simulink model "TST_CrCtl_Governor"  (R2016b)
settings: Solver=FixedStepDiscrete  StartTime=0.0  StopTime=simTime  FixedStep=sampleTime  RelTol=1e-3
values from neighbouring files (symbols this model uses):
  testCase = 1    [initTST_CrCtl_Governor_001.m]    (also in initTST_CrCtl_Governor_002.m = 2; initTST_CrCtl_Governor_003.m = 3; initTST_CrCtl_Governor_004.m = 4; initTST_CrCtl_Governor_005.m = 5)
libraries: simulink x144, UnitTest_Lib x110
(part 1 of 7)
settings Model: Creator=guanxiaoxing  LastModifiedBy=guanxiaoxing
settings DebuggingCC: SignalRangeChecking=error

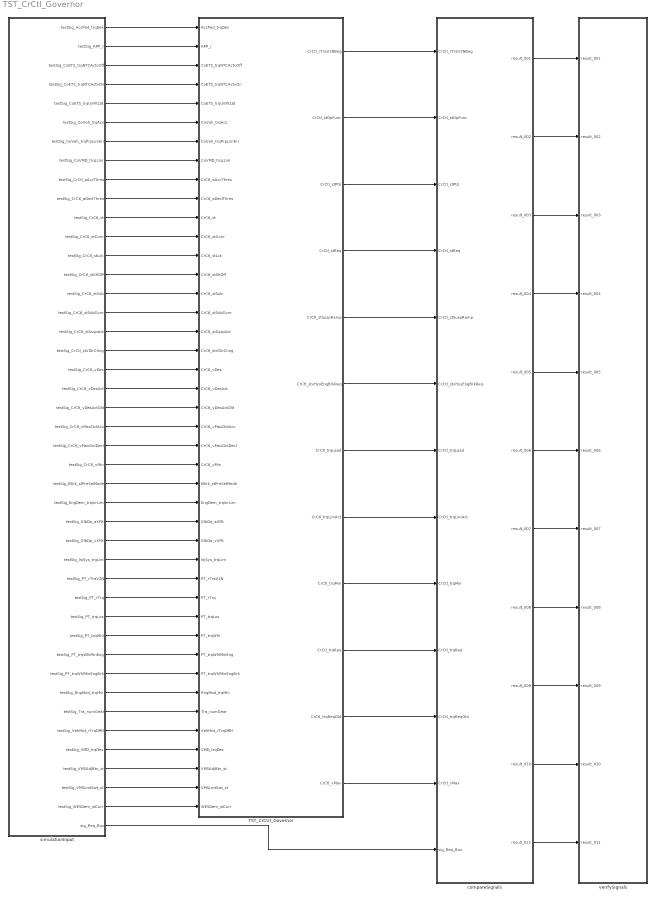
== system TST_CrCtl_Governor ==
  TST_CrCUI_Governor : Subsystem
  compareSignals : Subsystem
  simulationInput : Subsystem
  verifySignals : Subsystem
  wires:
  simulationInput/1(testSig_AccPed_trqDes) -> TST_CrCUI_Governor/1(AccPed_trqDes)
  simulationInput/2(testSig_APP_r) -> TST_CrCUI_Governor/2(APP_r)
  simulationInput/3(testSig_CoETS_trqNTCActvOff) -> TST_CrCUI_Governor/3(CoETS_trqNTCActvOff)
  simulationInput/4(testSig_CoETS_trqNTCActvOn) -> TST_CrCUI_Governor/4(CoETS_trqNTCActvOn)
  simulationInput/5(testSig_CoETS_trqUnFltLtd) -> TST_CrCUI_Governor/5(CoETS_trqUnFltLtd)
  simulationInput/6(testSig_CoVeh_trqAcs) -> TST_CrCUI_Governor/6(CoVeh_trqAcs)
  simulationInput/7(testSig_CoVeh_trqPrpLimErr) -> TST_CrCUI_Governor/7(CoVeh_trqPrpLimErr)
  simulationInput/8(testSig_CoVMD_trqLLim) -> TST_CrCUI_Governor/8(CoVMD_trqLLim)
  simulationInput/9(testSig_CrCtl_aAccThres) -> TST_CrCUI_Governor/9(CrCtl_aAccThres)
  simulationInput/10(testSig_CrCtl_aDeclThres) -> TST_CrCUI_Governor/10(CrCtl_aDeclThres)
  simulationInput/11(testSig_CrCtl_st) -> TST_CrCUI_Governor/11(CrCtl_st)
  simulationInput/12(testSig_CrCtl_stGvnr) -> TST_CrCUI_Governor/12(CrCtl_stGvnr)
  simulationInput/13(testSig_CrCtl_stLck) -> TST_CrCUI_Governor/13(CrCtl_stLck)
  simulationInput/14(testSig_CrCtl_stShOff) -> TST_CrCUI_Governor/14(CrCtl_stShOff)
  simulationInput/15(testSig_CrCtl_stSub) -> TST_CrCUI_Governor/15(CrCtl_stSub)
  simulationInput/16(testSig_CrCtl_stSubGvnr) -> TST_CrCUI_Governor/16(CrCtl_stSubGvnr)
  simulationInput/17(testSig_CrCtl_stSuspAct) -> TST_CrCUI_Governor/17(CrCtl_stSuspAct)
  simulationInput/18(testSig_CrCtl_stVDirChng) -> TST_CrCUI_Governor/18(CrCtl_stVDirChng)
  simulationInput/19(testSig_CrCtl_vDes) -> TST_CrCUI_Governor/19(CrCtl_vDes)
  simulationInput/20(testSig_CrCtl_vDesAct) -> TST_CrCUI_Governor/20(CrCtl_vDesAct)
  simulationInput/21(testSig_CrCtl_vDesActOld) -> TST_CrCUI_Governor/21(CrCtl_vDesActOld)
  simulationInput/22(testSig_CrCtl_vMaxDvtAcc) -> TST_CrCUI_Governor/22(CrCtl_vMaxDvtAcc)
  simulationInput/23(testSig_CrCtl_vMaxDvtDecl) -> TST_CrCUI_Governor/23(CrCtl_vMaxDvtDecl)
  simulationInput/24(testSig_CrCtl_vMin) -> TST_CrCUI_Governor/24(CrCtl_vMin)
  simulationInput/25(testSig_EBrk_stPreSelMode) -> TST_CrCUI_Governor/25(EBrk_stPreSelMode)
  simulationInput/26(testSig_EngDem_trqInrLim) -> TST_CrCUI_Governor/26(EngDem_trqInrLim)
  simulationInput/27(testSig_GlbDa_aXFlt) -> TST_CrCUI_Governor/27(GlbDa_aXFlt)
  simulationInput/28(testSig_GlbDa_vXFlt) -> TST_CrCUI_Governor/28(GlbDa_vXFlt)
  simulationInput/29(testSig_InjSys_trqLim) -> TST_CrCUI_Governor/29(InjSys_trqLim)
  simulationInput/30(testSig_PT_rTraV2N) -> TST_CrCUI_Governor/30(PT_rTraV2N)
  simulationInput/31(testSig_PT_rTrq) -> TST_CrCUI_Governor/31(PT_rTrq)
  simulationInput/32(testSig_PT_trqLos) -> TST_CrCUI_Governor/32(PT_trqLos)
  simulationInput/33(testSig_PT_trqWhl) -> TST_CrCUI_Governor/33(PT_trqWhl)
  simulationInput/34(testSig_PT_trqWhlMinEng) -> TST_CrCUI_Governor/34(PT_trqWhlMinEng)
  simulationInput/35(testSig_PT_trqWhlMinEngBrk) -> TST_CrCUI_Governor/35(PT_trqWhlMinEngBrk)
  simulationInput/36(testSig_RngMod_trqMin) -> TST_CrCUI_Governor/36(RngMod_trqMin)
  simulationInput/37(testSig_Tra_numGear) -> TST_CrCUI_Governor/37(Tra_numGear)
  simulationInput/38(testSig_VehMot_rTrqDfftl) -> TST_CrCUI_Governor/38(VehMot_rTrqDfftl)
  simulationInput/39(testSig_VMD_trqDes) -> TST_CrCUI_Governor/39(VMD_trqDes)
  simulationInput/40(testSig_VMSAdjBtn_st) -> TST_CrCUI_Governor/40(VMSAdjBtn_st)
  simulationInput/41(testSig_VMSLmtSwt_st) -> TST_CrCUI_Governor/41(VMSLmtSwt_st)
  simulationInput/42(testSig_WESDem_stCurr) -> TST_CrCUI_Governor/42(WESDem_stCurr)
  TST_CrCUI_Governor/1(CrCtl_rTraV2NBeg) -> compareSignals/1(CrCtl_rTraV2NBeg)
  TST_CrCUI_Governor/2(CrCtl_stOpFunc) -> compareSignals/2(CrCtl_stOpFunc)
  TST_CrCUI_Governor/3(CrCtl_stPtd) -> compareSignals/3(CrCtl_stPtd)
  TST_CrCUI_Governor/4(CrCtl_stReq) -> compareSignals/4(CrCtl_stReq)
  TST_CrCUI_Governor/5(CrCtl_stSuspRamp) -> compareSignals/5(CrCtl_stSuspRamp)
  TST_CrCUI_Governor/6(CrCtl_stvHysEngBrkReq) -> compareSignals/6(CrCtl_stvHysEngBrkReq)
  TST_CrCUI_Governor/7(CrCtl_trqLead) -> compareSignals/7(CrCtl_trqLead)
  TST_CrCUI_Governor/8(CrCtl_trqLimAct) -> compareSignals/8(CrCtl_trqLimAct)
  TST_CrCUI_Governor/9(CrCtl_trqMin) -> compareSignals/9(CrCtl_trqMin)
  TST_CrCUI_Governor/10(CrCtl_trqReq) -> compareSignals/10(CrCtl_trqReq)
  TST_CrCUI_Governor/11(CrCtl_trqReqOld) -> compareSignals/11(CrCtl_trqReqOld)
  TST_CrCUI_Governor/12(CrCtl_vMax) -> compareSignals/12(CrCtl_vMax)
  simulationInput/43(sig_Req_Bus) -> compareSignals/13(sig_Req_Bus)
  compareSignals/1(result_001) -> verifySignals/1(result_001)
  compareSignals/2(result_002) -> verifySignals/2(result_002)
  compareSignals/3(result_003) -> verifySignals/3(result_003)
  compareSignals/4(result_004) -> verifySignals/4(result_004)
  compareSignals/5(result_005) -> verifySignals/5(result_005)
  compareSignals/6(result_006) -> verifySignals/6(result_006)
  compareSignals/7(result_007) -> verifySignals/7(result_007)
  compareSignals/8(result_008) -> verifySignals/8(result_008)
  compareSignals/9(result_009) -> verifySignals/9(result_009)
  compareSignals/10(result_010) -> verifySignals/10(result_010)
  compareSignals/11(result_011) -> verifySignals/11(result_011)

== system TST_CrCtl_Governor/TST_CrCUI_Governor ==
  AccPed_trqDes : Inport
  APP_r : Inport  Port=2
  CoETS_trqNTCActvOff : Inport  Port=3
  CoETS_trqNTCActvOn : Inport  Port=4
  CoETS_trqUnFltLtd : Inport  Port=5
  CoVeh_trqAcs : Inport  Port=6
  CoVeh_trqPrpLimErr : Inport  Port=7
  CoVMD_trqLLim : Inport  Port=8
  CrCtl_aAccThres : Inport  Port=9
  CrCtl_aDeclThres : Inport  Port=10
  CrCtl_st : Inport  Port=11
  CrCtl_stGvnr : Inport  Port=12
  CrCtl_stLck : Inport  Port=13
  CrCtl_stShOff : Inport  Port=14
  CrCtl_stSub : Inport  Port=15
  CrCtl_stSubGvnr : Inport  Port=16
  CrCtl_stSuspAct : Inport  Port=17
  CrCtl_stVDirChng : Inport  Port=18
  CrCtl_vDes : Inport  Port=19
  CrCtl_vDesAct : Inport  Port=20
  CrCtl_vDesActOld : Inport  Port=21
  CrCtl_vMaxDvtAcc : Inport  Port=22
  CrCtl_vMaxDvtDecl : Inport  Port=23
  CrCtl_vMin : Inport  Port=24
  EBrk_stPreSelMode : Inport  Port=25
  EngDem_trqInrLim : Inport  Port=26
  GlbDa_aXFlt : Inport  Port=27
  GlbDa_vXFlt : Inport  Port=28
  InjSys_trqLim : Inport  Port=29
  PT_rTraV2N : Inport  Port=30
  PT_rTrq : Inport  Port=31
  PT_trqLos : Inport  Port=32
  PT_trqWhl : Inport  Port=33
  PT_trqWhlMinEng : Inport  Port=34
  PT_trqWhlMinEngBrk : Inport  Port=35
  RngMod_trqMin : Inport  Port=36
  Tra_numGear : Inport  Port=37
  VehMot_rTrqDfftl : Inport  Port=38
  VMD_trqDes : Inport  Port=39
  VMSAdjBtn_st : Inport  Port=40
  VMSLmtSwt_st : Inport  Port=41
  WESDem_stCurr : Inport  Port=42
  CrCUI_Governor : ModelReference  ModelNameDialog=CrCUI_Governor  SimulationMode=Normal  ModelReferenceVersion=1.278  TriggerPortName=function  TriggerPortTriggerType=function-call  TriggerPortStatesWhenEnabling=held
  Function_Call : simulink/Ports & Subsystems/Function-Call Generator  sample_time=sampleTime  numberOfIterations=1
  CrCtl_rTraV2NBeg : Outport
  CrCtl_stOpFunc : Outport  Port=2
  CrCtl_stPtd : Outport  Port=3
  CrCtl_stReq : Outport  Port=4
  CrCtl_stSuspRamp : Outport  Port=5
  CrCtl_stvHysEngBrkReq : Outport  Port=6
  CrCtl_trqLead : Outport  Port=7
  CrCtl_trqLimAct : Outport  Port=8
  CrCtl_trqMin : Outport  Port=9
  CrCtl_trqReq : Outport  Port=10
  CrCtl_trqReqOld : Outport  Port=11
  CrCtl_vMax : Outport  Port=12
  wires:
  Function_Call/1 -> CrCUI_Governor/Trigger
  AccPed_trqDes/1 -> CrCUI_Governor/1
  APP_r/1 -> CrCUI_Governor/2
  CoETS_trqNTCActvOff/1 -> CrCUI_Governor/3
  CoETS_trqNTCActvOn/1 -> CrCUI_Governor/4
  CoETS_trqUnFltLtd/1 -> CrCUI_Governor/5
  CoVeh_trqAcs/1 -> CrCUI_Governor/6
  CoVeh_trqPrpLimErr/1 -> CrCUI_Governor/7
  CoVMD_trqLLim/1 -> CrCUI_Governor/8
  CrCtl_aAccThres/1 -> CrCUI_Governor/9
  CrCtl_aDeclThres/1 -> CrCUI_Governor/10
  CrCtl_st/1 -> CrCUI_Governor/11
  CrCtl_stGvnr/1 -> CrCUI_Governor/12
  CrCtl_stLck/1 -> CrCUI_Governor/13
  CrCtl_stShOff/1 -> CrCUI_Governor/14
  CrCtl_stSub/1 -> CrCUI_Governor/15
  CrCtl_stSubGvnr/1 -> CrCUI_Governor/16
  CrCtl_stSuspAct/1 -> CrCUI_Governor/17
  CrCtl_stVDirChng/1 -> CrCUI_Governor/18
  CrCtl_vDes/1 -> CrCUI_Governor/19
  CrCtl_vDesAct/1 -> CrCUI_Governor/20
  CrCtl_vDesActOld/1 -> CrCUI_Governor/21
  CrCtl_vMaxDvtAcc/1 -> CrCUI_Governor/22
  CrCtl_vMaxDvtDecl/1 -> CrCUI_Governor/23
  CrCtl_vMin/1 -> CrCUI_Governor/24
  EBrk_stPreSelMode/1 -> CrCUI_Governor/25
  EngDem_trqInrLim/1 -> CrCUI_Governor/26
  GlbDa_aXFlt/1 -> CrCUI_Governor/27
  GlbDa_vXFlt/1 -> CrCUI_Governor/28
  InjSys_trqLim/1 -> CrCUI_Governor/29
  PT_rTraV2N/1 -> CrCUI_Governor/30
  PT_rTrq/1 -> CrCUI_Governor/31
  PT_trqLos/1 -> CrCUI_Governor/32
  PT_trqWhl/1 -> CrCUI_Governor/33
  PT_trqWhlMinEng/1 -> CrCUI_Governor/34
  PT_trqWhlMinEngBrk/1 -> CrCUI_Governor/35
  RngMod_trqMin/1 -> CrCUI_Governor/36
  Tra_numGear/1 -> CrCUI_Governor/37
  VehMot_rTrqDfftl/1 -> CrCUI_Governor/38
  VMD_trqDes/1 -> CrCUI_Governor/39
  VMSAdjBtn_st/1 -> CrCUI_Governor/40
  VMSLmtSwt_st/1 -> CrCUI_Governor/41
  WESDem_stCurr/1 -> CrCUI_Governor/42
  CrCUI_Governor/1 -> CrCtl_rTraV2NBeg/1
  CrCUI_Governor/2 -> CrCtl_stOpFunc/1
  CrCUI_Governor/3 -> CrCtl_stPtd/1
  CrCUI_Governor/4 -> CrCtl_stReq/1
  CrCUI_Governor/5 -> CrCtl_stSuspRamp/1
  CrCUI_Governor/6 -> CrCtl_stvHysEngBrkReq/1
  CrCUI_Governor/7 -> CrCtl_trqLead/1
  CrCUI_Governor/8 -> CrCtl_trqLimAct/1
  CrCUI_Governor/9 -> CrCtl_trqMin/1
  CrCUI_Governor/10 -> CrCtl_trqReq/1
  CrCUI_Governor/11 -> CrCtl_trqReqOld/1
  CrCUI_Governor/12 -> CrCtl_vMax/1

== system TST_CrCtl_Governor/compareSignals ==
  CrCtl_rTraV2NBeg : Inport
  CrCtl_stOpFunc : Inport  Port=2
  CrCtl_stPtd : Inport  Port=3
  CrCtl_stReq : Inport  Port=4
  CrCtl_stSuspRamp : Inport  Port=5
  CrCtl_stvHysEngBrkReq : Inport  Port=6
  CrCtl_trqLead : Inport  Port=7
  CrCtl_trqLimAct : Inport  Port=8
  CrCtl_trqMin : Inport  Port=9
  CrCtl_trqReq : Inport  Port=10
  CrCtl_trqReqOld : Inport  Port=11
  CrCtl_vMax : Inport  Port=12
  sig_Req_Bus : Inport  Port=13
  BC : BusCreator  Inputs=12
  CTC_001 : simulink/Logic and Bit Operations/Compare To Constant  relop===  const=1  OutDataTypeStr=boolean
  CTC_002 : simulink/Logic and Bit Operations/Compare To Constant  relop===  const=2  OutDataTypeStr=boolean
  CTC_003 : simulink/Logic and Bit Operations/Compare To Constant  relop===  const=3  OutDataTypeStr=boolean
  CTC_004 : simulink/Logic and Bit Operations/Compare To Constant  relop===  const=4  OutDataTypeStr=boolean
  CTC_005 : simulink/Logic and Bit Operations/Compare To Constant  relop===  const=5  OutDataTypeStr=boolean
  CTC_006 : simulink/Logic and Bit Operations/Compare To Constant  relop===  const=6  OutDataTypeStr=boolean
  CTC_007 : simulink/Logic and Bit Operations/Compare To Constant  relop===  const=7  OutDataTypeStr=boolean
  CTC_008 : simulink/Logic and Bit Operations/Compare To Constant  relop===  const=8  OutDataTypeStr=boolean
  CTC_009 : simulink/Logic and Bit Operations/Compare To Constant  relop===  const=9  OutDataTypeStr=boolean
  CTC_010 : simulink/Logic and Bit Operations/Compare To Constant  relop===  const=10  OutDataTypeStr=boolean
  CTC_011 : simulink/Logic and Bit Operations/Compare To Constant  relop===  const=11  OutDataTypeStr=boolean
  Requirement_001 : Subsystem
  Requirement_002 : Subsystem
  Requirement_003 : Subsystem
  Requirement_004 : Subsystem
  Requirement_005 : Subsystem
  Requirement_006 : Subsystem
  Requirement_007 : Subsystem
  Requirement_008 : Subsystem
  Requirement_009 : Subsystem
  Requirement_010 : Subsystem
  Requirement_011 : Subsystem
  TC_001 : Constant  Value=testCase
  TC_002 : Constant  Value=testCase
  TC_003 : Constant  Value=testCase
  TC_004 : Constant  Value=testCase
  TC_005 : Constant  Value=testCase
  TC_006 : Constant  Value=testCase
  TC_007 : Constant  Value=testCase
  TC_008 : Constant  Value=testCase
  TC_009 : Constant  Value=testCase
  TC_010 : Constant  Value=testCase
  TC_011 : Constant  Value=testCase
  result_001 : Outport
  result_002 : Outport  Port=2
  result_003 : Outport  Port=3
  result_004 : Outport  Port=4
  result_005 : Outport  Port=5
  result_006 : Outport  Port=6
  result_007 : Outport  Port=7
  result_008 : Outport  Port=8
  result_009 : Outport  Port=9
  result_010 : Outport  Port=10
  result_011 : Outport  Port=11
  wires:
  CrCtl_rTraV2NBeg/1 -> BC/1  "CrCtl_rTraV2NBeg"
  CrCtl_stOpFunc/1 -> BC/2  "CrCtl_stOpFunc"
  CrCtl_stPtd/1 -> BC/3  "CrCtl_stPtd"
  CrCtl_stReq/1 -> BC/4  "CrCtl_stReq"
  CrCtl_stSuspRamp/1 -> BC/5  "CrCtl_stSuspRamp"
  CrCtl_stvHysEngBrkReq/1 -> BC/6  "CrCtl_stvHysEngBrkReq"
  CrCtl_trqLead/1 -> BC/7  "CrCtl_trqLead"
  CrCtl_trqLimAct/1 -> BC/8  "CrCtl_trqLimAct"
  CrCtl_trqMin/1 -> BC/9  "CrCtl_trqMin"
  CrCtl_trqReq/1 -> BC/10  "CrCtl_trqReq"
  CrCtl_trqReqOld/1 -> BC/11  "CrCtl_trqReqOld"
  CrCtl_vMax/1 -> BC/12  "CrCtl_vMax"
  TC_001/1 -> CTC_001/1
  CTC_001/1 -> Requirement_001/Enable
  sig_Req_Bus/1 -> Requirement_010/2(sig_Req_Bus), Requirement_011/2(sig_Req_Bus), Requirement_009/2(sig_Req_Bus), Requirement_008/2(sig_Req_Bus), Requirement_007/2(sig_Req_Bus), Requirement_006/2(sig_Req_Bus), Requirement_005/2(sig_Req_Bus), Requirement_004/2(sig_Req_Bus), Requirement_001/2(sig_Req_Bus), Requirement_002/2(sig_Req_Bus), Requirement_003/2(sig_Req_Bus)
  BC/1 -> Requirement_010/1(sig_Result_Bus), Requirement_011/1(sig_Result_Bus), Requirement_009/1(sig_Result_Bus), Requirement_008/1(sig_Result_Bus), Requirement_007/1(sig_Result_Bus), Requirement_006/1(sig_Result_Bus), Requirement_005/1(sig_Result_Bus), Requirement_004/1(sig_Result_Bus), Requirement_003/1(sig_Result_Bus), Requirement_002/1(sig_Result_Bus), Requirement_001/1(sig_Result_Bus)
  Requirement_001/1(result) -> result_001/1
  TC_002/1 -> CTC_002/1
  CTC_002/1 -> Requirement_002/Enable
  Requirement_002/1(result) -> result_002/1
  TC_003/1 -> CTC_003/1
  CTC_003/1 -> Requirement_003/Enable
  Requirement_003/1(result) -> result_003/1
  TC_004/1 -> CTC_004/1
  CTC_004/1 -> Requirement_004/Enable
  Requirement_004/1(result) -> result_004/1
  TC_005/1 -> CTC_005/1
  CTC_005/1 -> Requirement_005/Enable
  Requirement_005/1(result) -> result_005/1
  TC_006/1 -> CTC_006/1
  CTC_006/1 -> Requirement_006/Enable
  Requirement_006/1(result) -> result_006/1
  TC_007/1 -> CTC_007/1
  CTC_007/1 -> Requirement_007/Enable
  Requirement_007/1(result) -> result_007/1
  TC_008/1 -> CTC_008/1
  CTC_008/1 -> Requirement_008/Enable
  Requirement_008/1(result) -> result_008/1
  TC_009/1 -> CTC_009/1
  CTC_009/1 -> Requirement_009/Enable
  Requirement_009/1(result) -> result_009/1
  TC_010/1 -> CTC_010/1
  CTC_010/1 -> Requirement_010/Enable
  Requirement_010/1(result) -> result_010/1
  TC_011/1 -> CTC_011/1
  CTC_011/1 -> Requirement_011/Enable
  Requirement_011/1(result) -> result_011/1

== system TST_CrCtl_Governor/simulationInput ==
  BS : BusSelector  OutputSignals=testSig_AccPed_trqDes,testSig_APP_r,testSig_CoETS_trqNTCActvOff,testSig_CoETS_trqNTCActvOn,testSig_CoETS_trqUnFltLtd,testSig_CoVeh_trqAcs,testSig_CoVeh_trqPrpLimErr,testSig_CoVMD_trqLLim,testSig_CrCtl_aAccThres,testSig_CrCtl_aDeclThres,testSig_CrCtl_st,testSig_CrCtl_stGvnr,testSig_CrCtl_stLck,testSig_CrCtl_stShOff,testSig_CrCtl_stSub,testSig_CrCtl_stSubGvnr,testSig_CrCtl_stSuspAct,testSig_CrCtl_stVDirChng,testSig_CrCtl_vDes,testSig_CrCtl_vDesAct,testSig_CrCtl_vDesActOld,testSig_CrCtl_vMaxDvtAcc,testSig_CrCtl_vMaxDvtDecl,testSig_CrCtl_vMin,testSig_EBrk_stPreSelMode,testSig_EngDem_trqInrLim,testSig_GlbDa_aXFlt,testSig_GlbDa_vXFlt,testSig_InjSys_trqLim,testSig_PT_rTraV2N,testSig_PT_rTrq,testSig_PT_trqLos,testSig_PT_trqWhl,testSig_PT_trqWhlMinEng,testSig_PT_trqWhlMinEngBrk,testSig_RngMod_trqMin,testSig_Tra_numGear,testSig_VehMot_rTrqDfftl,testSig_VMD_trqDes,testSig_VMSAdjBtn_st,testSig_VMSLmtSwt_st,testSig_WESDem_stCurr
  MPSw : MultiPortSwitch  Inputs=11  SaturateOnIntegerOverflow=on  InputSameDT=on
  TestCase : Constant  Value=testCase
  testSignals_R001 : Subsystem
  testSignals_R002 : Subsystem
  testSignals_R003 : Subsystem
  testSignals_R004 : Subsystem
  testSignals_R005 : Subsystem
  testSignals_R006 : Subsystem
  testSignals_R007 : Subsystem
  testSignals_R008 : Subsystem
  testSignals_R009 : Subsystem
  testSignals_R010 : Subsystem
  testSignals_R011 : Subsystem
  testSig_AccPed_trqDes : Outport
  testSig_APP_r : Outport  Port=2
  testSig_CoETS_trqNTCActvOff : Outport  Port=3
  testSig_CoETS_trqNTCActvOn : Outport  Port=4
  testSig_CoETS_trqUnFltLtd : Outport  Port=5
  testSig_CoVeh_trqAcs : Outport  Port=6
  testSig_CoVeh_trqPrpLimErr : Outport  Port=7
  testSig_CoVMD_trqLLim : Outport  Port=8
  testSig_CrCtl_aAccThres : Outport  Port=9
  testSig_CrCtl_aDeclThres : Outport  Port=10
  testSig_CrCtl_st : Outport  Port=11
  testSig_CrCtl_stGvnr : Outport  Port=12
  testSig_CrCtl_stLck : Outport  Port=13
  testSig_CrCtl_stShOff : Outport  Port=14
  testSig_CrCtl_stSub : Outport  Port=15
  testSig_CrCtl_stSubGvnr : Outport  Port=16
  testSig_CrCtl_stSuspAct : Outport  Port=17
  testSig_CrCtl_stVDirChng : Outport  Port=18
  testSig_CrCtl_vDes : Outport  Port=19
  testSig_CrCtl_vDesAct : Outport  Port=20
  testSig_CrCtl_vDesActOld : Outport  Port=21
  testSig_CrCtl_vMaxDvtAcc : Outport  Port=22
  testSig_CrCtl_vMaxDvtDecl : Outport  Port=23
  testSig_CrCtl_vMin : Outport  Port=24
  testSig_EBrk_stPreSelMode : Outport  Port=25
  testSig_EngDem_trqInrLim : Outport  Port=26
  testSig_GlbDa_aXFlt : Outport  Port=27
  testSig_GlbDa_vXFlt : Outport  Port=28
  testSig_InjSys_trqLim : Outport  Port=29
  testSig_PT_rTraV2N : Outport  Port=30
  testSig_PT_rTrq : Outport  Port=31
  testSig_PT_trqLos : Outport  Port=32
  testSig_PT_trqWhl : Outport  Port=33
  testSig_PT_trqWhlMinEng : Outport  Port=34
  testSig_PT_trqWhlMinEngBrk : Outport  Port=35
  testSig_RngMod_trqMin : Outport  Port=36
  testSig_Tra_numGear : Outport  Port=37
  testSig_VehMot_rTrqDfftl : Outport  Port=38
  testSig_VMD_trqDes : Outport  Port=39
  testSig_VMSAdjBtn_st : Outport  Port=40
  testSig_VMSLmtSwt_st : Outport  Port=41
  testSig_WESDem_stCurr : Outport  Port=42
  sig_Req_Bus : Outport  Port=43
  wires:
  BS/1 -> testSig_AccPed_trqDes/1  "<testSig_AccPed_trqDes>"
  BS/2 -> testSig_APP_r/1  "<testSig_APP_r>"
  BS/3 -> testSig_CoETS_trqNTCActvOff/1  "<testSig_CoETS_trqNTCActvOff>"
  BS/4 -> testSig_CoETS_trqNTCActvOn/1  "<testSig_CoETS_trqNTCActvOn>"
  BS/5 -> testSig_CoETS_trqUnFltLtd/1  "<testSig_CoETS_trqUnFltLtd>"
  BS/6 -> testSig_CoVeh_trqAcs/1  "<testSig_CoVeh_trqAcs>"
  BS/7 -> testSig_CoVeh_trqPrpLimErr/1  "<testSig_CoVeh_trqPrpLimErr>"
  BS/8 -> testSig_CoVMD_trqLLim/1  "<testSig_CoVMD_trqLLim>"
  BS/9 -> testSig_CrCtl_aAccThres/1  "<testSig_CrCtl_aAccThres>"
  BS/10 -> testSig_CrCtl_aDeclThres/1  "<testSig_CrCtl_aDeclThres>"
  BS/11 -> testSig_CrCtl_st/1  "<testSig_CrCtl_st>"
  BS/12 -> testSig_CrCtl_stGvnr/1  "<testSig_CrCtl_stGvnr>"
  BS/13 -> testSig_CrCtl_stLck/1  "<testSig_CrCtl_stLck>"
  BS/14 -> testSig_CrCtl_stShOff/1  "<testSig_CrCtl_stShOff>"
  BS/15 -> testSig_CrCtl_stSub/1  "<testSig_CrCtl_stSub>"
  BS/16 -> testSig_CrCtl_stSubGvnr/1  "<testSig_CrCtl_stSubGvnr>"
  BS/17 -> testSig_CrCtl_stSuspAct/1  "<testSig_CrCtl_stSuspAct>"
  BS/18 -> testSig_CrCtl_stVDirChng/1  "<testSig_CrCtl_stVDirChng>"
  BS/19 -> testSig_CrCtl_vDes/1  "<testSig_CrCtl_vDes>"
  BS/20 -> testSig_CrCtl_vDesAct/1  "<testSig_CrCtl_vDesAct>"
  BS/21 -> testSig_CrCtl_vDesActOld/1  "<testSig_CrCtl_vDesActOld>"
  BS/22 -> testSig_CrCtl_vMaxDvtAcc/1  "<testSig_CrCtl_vMaxDvtAcc>"
  BS/23 -> testSig_CrCtl_vMaxDvtDecl/1  "<testSig_CrCtl_vMaxDvtDecl>"
  BS/24 -> testSig_CrCtl_vMin/1  "<testSig_CrCtl_vMin>"
  BS/25 -> testSig_EBrk_stPreSelMode/1  "<testSig_EBrk_stPreSelMode>"
  BS/26 -> testSig_EngDem_trqInrLim/1  "<testSig_EngDem_trqInrLim>"
  BS/27 -> testSig_GlbDa_aXFlt/1  "<testSig_GlbDa_aXFlt>"
  BS/28 -> testSig_GlbDa_vXFlt/1  "<testSig_GlbDa_vXFlt>"
  BS/29 -> testSig_InjSys_trqLim/1  "<testSig_InjSys_trqLim>"
  BS/30 -> testSig_PT_rTraV2N/1  "<testSig_PT_rTraV2N>"
  BS/31 -> testSig_PT_rTrq/1  "<testSig_PT_rTrq>"
  BS/32 -> testSig_PT_trqLos/1  "<testSig_PT_trqLos>"
  BS/33 -> testSig_PT_trqWhl/1  "<testSig_PT_trqWhl>"
  BS/34 -> testSig_PT_trqWhlMinEng/1  "<testSig_PT_trqWhlMinEng>"
  BS/35 -> testSig_PT_trqWhlMinEngBrk/1  "<testSig_PT_trqWhlMinEngBrk>"
  BS/36 -> testSig_RngMod_trqMin/1  "<testSig_RngMod_trqMin>"
  BS/37 -> testSig_Tra_numGear/1  "<testSig_Tra_numGear>"
  BS/38 -> testSig_VehMot_rTrqDfftl/1  "<testSig_VehMot_rTrqDfftl>"
  BS/39 -> testSig_VMD_trqDes/1  "<testSig_VMD_trqDes>"
  BS/40 -> testSig_VMSAdjBtn_st/1  "<testSig_VMSAdjBtn_st>"
  BS/41 -> testSig_VMSLmtSwt_st/1  "<testSig_VMSLmtSwt_st>"
  BS/42 -> testSig_WESDem_stCurr/1  "<testSig_WESDem_stCurr>"
  MPSw/1 -> BS/1, sig_Req_Bus/1
  TestCase/1 -> MPSw/1
  testSignals_R001/1(testSignals) -> MPSw/2
  testSignals_R002/1(testSignals) -> MPSw/3
  testSignals_R003/1(testSignals) -> MPSw/4
  testSignals_R004/1(testSignals) -> MPSw/5
  testSignals_R005/1(testSignals) -> MPSw/6
  testSignals_R006/1(testSignals) -> MPSw/7
  testSignals_R007/1(testSignals) -> MPSw/8
  testSignals_R008/1(testSignals) -> MPSw/9
  testSignals_R009/1(testSignals) -> MPSw/10
  testSignals_R010/1(testSignals) -> MPSw/11
  testSignals_R011/1(testSignals) -> MPSw/12

== system TST_CrCtl_Governor/verifySignals ==
  result_001 : Inport
  result_002 : Inport  Port=2
  result_003 : Inport  Port=3
  result_004 : Inport  Port=4
  result_005 : Inport  Port=5
  result_006 : Inport  Port=6
  result_007 : Inport  Port=7
  result_008 : Inport  Port=8
  result_009 : Inport  Port=9
  result_010 : Inport  Port=10
  result_011 : Inport  Port=11
  Assertion_001 : Assertion  Enabled=off
  Assertion_002 : Assertion  Enabled=off
  Assertion_003 : Assertion  Enabled=off
  Assertion_004 : Assertion  Enabled=off
  Assertion_005 : Assertion  Enabled=off
  Assertion_006 : Assertion  Enabled=off
  Assertion_007 : Assertion  Enabled=off
  Assertion_008 : Assertion  Enabled=off
  Assertion_009 : Assertion  Enabled=off
  Assertion_010 : Assertion  Enabled=off
  Assertion_011 : Assertion  Enabled=off
  wires:
  result_001/1 -> Assertion_001/1
  result_002/1 -> Assertion_002/1
  result_003/1 -> Assertion_003/1
  result_004/1 -> Assertion_004/1
  result_005/1 -> Assertion_005/1
  result_006/1 -> Assertion_006/1
  result_007/1 -> Assertion_007/1
  result_008/1 -> Assertion_008/1
  result_009/1 -> Assertion_009/1
  result_010/1 -> Assertion_010/1
  result_011/1 -> Assertion_011/1

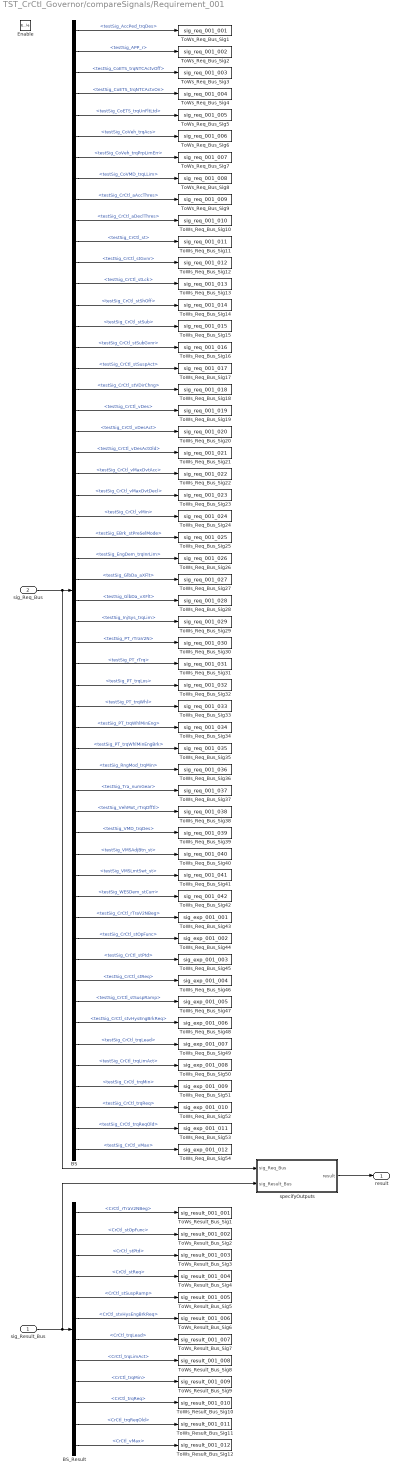
== system TST_CrCtl_Governor/compareSignals/Requirement_001 ==
  sig_Result_Bus : Inport
  sig_Req_Bus : Inport  Port=2
  Enable : EnablePort
  BS : BusSelector  OutputSignals=testSig_AccPed_trqDes,testSig_APP_r,testSig_CoETS_trqNTCActvOff,testSig_CoETS_trqNTCActvOn,testSig_CoETS_trqUnFltLtd,testSig_CoVeh_trqAcs,testSig_CoVeh_trqPrpLimErr,testSig_CoVMD_trqLLim,testSig_CrCtl_aAccThres,testSig_CrCtl_aDeclThres,testSig_CrCtl_st,testSig_CrCtl_stGvnr,testSig_CrCtl_stLck,testSig_CrCtl_stShOff,testSig_CrCtl_stSub,testSig_CrCtl_stSubGvnr,testSig_CrCtl_stSuspAct,testSig_CrCtl_stVDirChng,testSig_CrCtl_vDes,testSig_CrCtl_vDesAct,testSig_CrCtl_vDesActOld,testSig_CrCtl_vMaxDvtAcc,testSig_CrCtl_vMaxDvtDecl,testSig_CrCtl_vMin,testSig_EBrk_stPreSelMode,testSig_EngDem_trqInrLim,testSig_GlbDa_aXFlt,testSig_GlbDa_vXFlt,testSig_InjSys_trqLim,testSig_PT_rTraV2N,testSig_PT_rTrq,testSig_PT_trqLos,testSig_PT_trqWhl,testSig_PT_trqWhlMinEng,testSig_PT_trqWhlMinEngBrk,testSig_RngMod_trqMin,testSig_Tra_numGear,testSig_VehMot_rTrqDfftl,testSig_VMD_trqDes,testSig_VMSAdjBtn_st,testSig_VMSLmtSwt_st,testSig_WESDem_stCurr,testSig_CrCtl_rTraV2NBeg,testSig_CrCtl_stOpFunc,testSig_CrCtl_stPtd,testSig_CrCtl_stReq,testSig_CrCtl_stSuspRamp,testSig_CrCtl_stvHysEngBrkReq,testSig_CrCtl_trqLead,testSig_CrCtl_trqLimAct,testSig_CrCtl_trqMin,testSig_CrCtl_trqReq,testSig_CrCtl_trqReqOld,testSig_CrCtl_vMax
  BS_Result : BusSelector  OutputSignals=CrCtl_rTraV2NBeg,CrCtl_stOpFunc,CrCtl_stPtd,CrCtl_stReq,CrCtl_stSuspRamp,CrCtl_stvHysEngBrkReq,CrCtl_trqLead,CrCtl_trqLimAct,CrCtl_trqMin,CrCtl_trqReq,CrCtl_trqReqOld,CrCtl_vMax
  ToWs_Req_Bus_Sig1 : ToWorkspace  VariableName=sig_req_001_001  SaveFormat=Structure With Time
  ToWs_Req_Bus_Sig10 : ToWorkspace  VariableName=sig_req_001_010  SaveFormat=Structure With Time
  ToWs_Req_Bus_Sig11 : ToWorkspace  VariableName=sig_req_001_011  SaveFormat=Structure With Time
  ToWs_Req_Bus_Sig12 : ToWorkspace  VariableName=sig_req_001_012  SaveFormat=Structure With Time
  ToWs_Req_Bus_Sig13 : ToWorkspace  VariableName=sig_req_001_013  SaveFormat=Structure With Time
  ToWs_Req_Bus_Sig14 : ToWorkspace  VariableName=sig_req_001_014  SaveFormat=Structure With Time
  ToWs_Req_Bus_Sig15 : ToWorkspace  VariableName=sig_req_001_015  SaveFormat=Structure With Time
  ToWs_Req_Bus_Sig16 : ToWorkspace  VariableName=sig_req_001_016  SaveFormat=Structure With Time
  ToWs_Req_Bus_Sig17 : ToWorkspace  VariableName=sig_req_001_017  SaveFormat=Structure With Time
  ToWs_Req_Bus_Sig18 : ToWorkspace  VariableName=sig_req_001_018  SaveFormat=Structure With Time
  ToWs_Req_Bus_Sig19 : ToWorkspace  VariableName=sig_req_001_019  SaveFormat=Structure With Time
  ToWs_Req_Bus_Sig2 : ToWorkspace  VariableName=sig_req_001_002  SaveFormat=Structure With Time
  ToWs_Req_Bus_Sig20 : ToWorkspace  VariableName=sig_req_001_020  SaveFormat=Structure With Time
  ToWs_Req_Bus_Sig21 : ToWorkspace  VariableName=sig_req_001_021  SaveFormat=Structure With Time
  ToWs_Req_Bus_Sig22 : ToWorkspace  VariableName=sig_req_001_022  SaveFormat=Structure With Time
  ToWs_Req_Bus_Sig23 : ToWorkspace  VariableName=sig_req_001_023  SaveFormat=Structure With Time
  ToWs_Req_Bus_Sig24 : ToWorkspace  VariableName=sig_req_001_024  SaveFormat=Structure With Time
  ToWs_Req_Bus_Sig25 : ToWorkspace  VariableName=sig_req_001_025  SaveFormat=Structure With Time
  ToWs_Req_Bus_Sig26 : ToWorkspace  VariableName=sig_req_001_026  SaveFormat=Structure With Time
  ToWs_Req_Bus_Sig27 : ToWorkspace  VariableName=sig_req_001_027  SaveFormat=Structure With Time
  ToWs_Req_Bus_Sig28 : ToWorkspace  VariableName=sig_req_001_028  SaveFormat=Structure With Time
  ToWs_Req_Bus_Sig29 : ToWorkspace  VariableName=sig_req_001_029  SaveFormat=Structure With Time
  ToWs_Req_Bus_Sig3 : ToWorkspace  VariableName=sig_req_001_003  SaveFormat=Structure With Time
  ToWs_Req_Bus_Sig30 : ToWorkspace  VariableName=sig_req_001_030  SaveFormat=Structure With Time
  ToWs_Req_Bus_Sig31 : ToWorkspace  VariableName=sig_req_001_031  SaveFormat=Structure With Time
  ToWs_Req_Bus_Sig32 : ToWorkspace  VariableName=sig_req_001_032  SaveFormat=Structure With Time
  ToWs_Req_Bus_Sig33 : ToWorkspace  VariableName=sig_req_001_033  SaveFormat=Structure With Time
  ToWs_Req_Bus_Sig34 : ToWorkspace  VariableName=sig_req_001_034  SaveFormat=Structure With Time
  ToWs_Req_Bus_Sig35 : ToWorkspace  VariableName=sig_req_001_035  SaveFormat=Structure With Time
  ToWs_Req_Bus_Sig36 : ToWorkspace  VariableName=sig_req_001_036  SaveFormat=Structure With Time
  ToWs_Req_Bus_Sig37 : ToWorkspace  VariableName=sig_req_001_037  SaveFormat=Structure With Time
  ToWs_Req_Bus_Sig38 : ToWorkspace  VariableName=sig_req_001_038  SaveFormat=Structure With Time
  ToWs_Req_Bus_Sig39 : ToWorkspace  VariableName=sig_req_001_039  SaveFormat=Structure With Time
  ToWs_Req_Bus_Sig4 : ToWorkspace  VariableName=sig_req_001_004  SaveFormat=Structure With Time
  ToWs_Req_Bus_Sig40 : ToWorkspace  VariableName=sig_req_001_040  SaveFormat=Structure With Time
  ToWs_Req_Bus_Sig41 : ToWorkspace  VariableName=sig_req_001_041  SaveFormat=Structure With Time
  ToWs_Req_Bus_Sig42 : ToWorkspace  VariableName=sig_req_001_042  SaveFormat=Structure With Time
  ToWs_Req_Bus_Sig43 : ToWorkspace  VariableName=sig_exp_001_001  SaveFormat=Structure With Time
  ToWs_Req_Bus_Sig44 : ToWorkspace  VariableName=sig_exp_001_002  SaveFormat=Structure With Time
  ToWs_Req_Bus_Sig45 : ToWorkspace  VariableName=sig_exp_001_003  SaveFormat=Structure With Time
  ToWs_Req_Bus_Sig46 : ToWorkspace  VariableName=sig_exp_001_004  SaveFormat=Structure With Time
  ToWs_Req_Bus_Sig47 : ToWorkspace  VariableName=sig_exp_001_005  SaveFormat=Structure With Time
  ToWs_Req_Bus_Sig48 : ToWorkspace  VariableName=sig_exp_001_006  SaveFormat=Structure With Time
  ToWs_Req_Bus_Sig49 : ToWorkspace  VariableName=sig_exp_001_007  SaveFormat=Structure With Time
  ToWs_Req_Bus_Sig5 : ToWorkspace  VariableName=sig_req_001_005  SaveFormat=Structure With Time
  ToWs_Req_Bus_Sig50 : ToWorkspace  VariableName=sig_exp_001_008  SaveFormat=Structure With Time
  ToWs_Req_Bus_Sig51 : ToWorkspace  VariableName=sig_exp_001_009  SaveFormat=Structure With Time
  ToWs_Req_Bus_Sig52 : ToWorkspace  VariableName=sig_exp_001_010  SaveFormat=Structure With Time
  ToWs_Req_Bus_Sig53 : ToWorkspace  VariableName=sig_exp_001_011  SaveFormat=Structure With Time
  ToWs_Req_Bus_Sig54 : ToWorkspace  VariableName=sig_exp_001_012  SaveFormat=Structure With Time
  ToWs_Req_Bus_Sig6 : ToWorkspace  VariableName=sig_req_001_006  SaveFormat=Structure With Time
  ToWs_Req_Bus_Sig7 : ToWorkspace  VariableName=sig_req_001_007  SaveFormat=Structure With Time
  ToWs_Req_Bus_Sig8 : ToWorkspace  VariableName=sig_req_001_008  SaveFormat=Structure With Time
  ToWs_Req_Bus_Sig9 : ToWorkspace  VariableName=sig_req_001_009  SaveFormat=Structure With Time
  ToWs_Result_Bus_Sig1 : ToWorkspace  VariableName=sig_result_001_001  SaveFormat=Structure With Time
  ToWs_Result_Bus_Sig10 : ToWorkspace  VariableName=sig_result_001_010  SaveFormat=Structure With Time
  ToWs_Result_Bus_Sig11 : ToWorkspace  VariableName=sig_result_001_011  SaveFormat=Structure With Time
  ToWs_Result_Bus_Sig12 : ToWorkspace  VariableName=sig_result_001_012  SaveFormat=Structure With Time
  ToWs_Result_Bus_Sig2 : ToWorkspace  VariableName=sig_result_001_002  SaveFormat=Structure With Time
  ToWs_Result_Bus_Sig3 : ToWorkspace  VariableName=sig_result_001_003  SaveFormat=Structure With Time
  ToWs_Result_Bus_Sig4 : ToWorkspace  VariableName=sig_result_001_004  SaveFormat=Structure With Time
  ToWs_Result_Bus_Sig5 : ToWorkspace  VariableName=sig_result_001_005  SaveFormat=Structure With Time
  ToWs_Result_Bus_Sig6 : ToWorkspace  VariableName=sig_result_001_006  SaveFormat=Structure With Time
  ToWs_Result_Bus_Sig7 : ToWorkspace  VariableName=sig_result_001_007  SaveFormat=Structure With Time
  ToWs_Result_Bus_Sig8 : ToWorkspace  VariableName=sig_result_001_008  SaveFormat=Structure With Time
  ToWs_Result_Bus_Sig9 : ToWorkspace  VariableName=sig_result_001_009  SaveFormat=Structure With Time
  specifyOutputs : Subsystem
  result : Outport
  wires:
  sig_Req_Bus/1 -> BS/1, specifyOutputs/1(sig_Req_Bus)
  BS/1 -> ToWs_Req_Bus_Sig1/1  "<testSig_AccPed_trqDes>"
  BS/2 -> ToWs_Req_Bus_Sig2/1  "<testSig_APP_r>"
  BS/3 -> ToWs_Req_Bus_Sig3/1  "<testSig_CoETS_trqNTCActvOff>"
  BS/4 -> ToWs_Req_Bus_Sig4/1  "<testSig_CoETS_trqNTCActvOn>"
  BS/5 -> ToWs_Req_Bus_Sig5/1  "<testSig_CoETS_trqUnFltLtd>"
  BS/6 -> ToWs_Req_Bus_Sig6/1  "<testSig_CoVeh_trqAcs>"
  BS/7 -> ToWs_Req_Bus_Sig7/1  "<testSig_CoVeh_trqPrpLimErr>"
  BS/8 -> ToWs_Req_Bus_Sig8/1  "<testSig_CoVMD_trqLLim>"
  BS/9 -> ToWs_Req_Bus_Sig9/1  "<testSig_CrCtl_aAccThres>"
  BS/10 -> ToWs_Req_Bus_Sig10/1  "<testSig_CrCtl_aDeclThres>"
  BS/11 -> ToWs_Req_Bus_Sig11/1  "<testSig_CrCtl_st>"
  BS/12 -> ToWs_Req_Bus_Sig12/1  "<testSig_CrCtl_stGvnr>"
  BS/13 -> ToWs_Req_Bus_Sig13/1  "<testSig_CrCtl_stLck>"
  BS/14 -> ToWs_Req_Bus_Sig14/1  "<testSig_CrCtl_stShOff>"
  BS/15 -> ToWs_Req_Bus_Sig15/1  "<testSig_CrCtl_stSub>"
  BS/16 -> ToWs_Req_Bus_Sig16/1  "<testSig_CrCtl_stSubGvnr>"
  BS/17 -> ToWs_Req_Bus_Sig17/1  "<testSig_CrCtl_stSuspAct>"
  BS/18 -> ToWs_Req_Bus_Sig18/1  "<testSig_CrCtl_stVDirChng>"
  BS/19 -> ToWs_Req_Bus_Sig19/1  "<testSig_CrCtl_vDes>"
  BS/20 -> ToWs_Req_Bus_Sig20/1  "<testSig_CrCtl_vDesAct>"
  BS/21 -> ToWs_Req_Bus_Sig21/1  "<testSig_CrCtl_vDesActOld>"
  BS/22 -> ToWs_Req_Bus_Sig22/1  "<testSig_CrCtl_vMaxDvtAcc>"
  BS/23 -> ToWs_Req_Bus_Sig23/1  "<testSig_CrCtl_vMaxDvtDecl>"
  BS/24 -> ToWs_Req_Bus_Sig24/1  "<testSig_CrCtl_vMin>"
  BS/25 -> ToWs_Req_Bus_Sig25/1  "<testSig_EBrk_stPreSelMode>"
  BS/26 -> ToWs_Req_Bus_Sig26/1  "<testSig_EngDem_trqInrLim>"
  BS/27 -> ToWs_Req_Bus_Sig27/1  "<testSig_GlbDa_aXFlt>"
  BS/28 -> ToWs_Req_Bus_Sig28/1  "<testSig_GlbDa_vXFlt>"
  BS/29 -> ToWs_Req_Bus_Sig29/1  "<testSig_InjSys_trqLim>"
  BS/30 -> ToWs_Req_Bus_Sig30/1  "<testSig_PT_rTraV2N>"
  BS/31 -> ToWs_Req_Bus_Sig31/1  "<testSig_PT_rTrq>"
  BS/32 -> ToWs_Req_Bus_Sig32/1  "<testSig_PT_trqLos>"
  BS/33 -> ToWs_Req_Bus_Sig33/1  "<testSig_PT_trqWhl>"
  BS/34 -> ToWs_Req_Bus_Sig34/1  "<testSig_PT_trqWhlMinEng>"
  BS/35 -> ToWs_Req_Bus_Sig35/1  "<testSig_PT_trqWhlMinEngBrk>"
  BS/36 -> ToWs_Req_Bus_Sig36/1  "<testSig_RngMod_trqMin>"
  BS/37 -> ToWs_Req_Bus_Sig37/1  "<testSig_Tra_numGear>"
  BS/38 -> ToWs_Req_Bus_Sig38/1  "<testSig_VehMot_rTrqDfftl>"
  BS/39 -> ToWs_Req_Bus_Sig39/1  "<testSig_VMD_trqDes>"
  BS/40 -> ToWs_Req_Bus_Sig40/1  "<testSig_VMSAdjBtn_st>"
  BS/41 -> ToWs_Req_Bus_Sig41/1  "<testSig_VMSLmtSwt_st>"
  BS/42 -> ToWs_Req_Bus_Sig42/1  "<testSig_WESDem_stCurr>"
  BS/43 -> ToWs_Req_Bus_Sig43/1  "<testSig_CrCtl_rTraV2NBeg>"
  BS/44 -> ToWs_Req_Bus_Sig44/1  "<testSig_CrCtl_stOpFunc>"
  BS/45 -> ToWs_Req_Bus_Sig45/1  "<testSig_CrCtl_stPtd>"
  BS/46 -> ToWs_Req_Bus_Sig46/1  "<testSig_CrCtl_stReq>"
  BS/47 -> ToWs_Req_Bus_Sig47/1  "<testSig_CrCtl_stSuspRamp>"
  BS/48 -> ToWs_Req_Bus_Sig48/1  "<testSig_CrCtl_stvHysEngBrkReq>"
  BS/49 -> ToWs_Req_Bus_Sig49/1  "<testSig_CrCtl_trqLead>"
  BS/50 -> ToWs_Req_Bus_Sig50/1  "<testSig_CrCtl_trqLimAct>"
  BS/51 -> ToWs_Req_Bus_Sig51/1  "<testSig_CrCtl_trqMin>"
  BS/52 -> ToWs_Req_Bus_Sig52/1  "<testSig_CrCtl_trqReq>"
  BS/53 -> ToWs_Req_Bus_Sig53/1  "<testSig_CrCtl_trqReqOld>"
  BS/54 -> ToWs_Req_Bus_Sig54/1  "<testSig_CrCtl_vMax>"
  sig_Result_Bus/1 -> BS_Result/1, specifyOutputs/2(sig_Result_Bus)
  BS_Result/1 -> ToWs_Result_Bus_Sig1/1  "<CrCtl_rTraV2NBeg>"
  BS_Result/2 -> ToWs_Result_Bus_Sig2/1  "<CrCtl_stOpFunc>"
  BS_Result/3 -> ToWs_Result_Bus_Sig3/1  "<CrCtl_stPtd>"
  BS_Result/4 -> ToWs_Result_Bus_Sig4/1  "<CrCtl_stReq>"
  BS_Result/5 -> ToWs_Result_Bus_Sig5/1  "<CrCtl_stSuspRamp>"
  BS_Result/6 -> ToWs_Result_Bus_Sig6/1  "<CrCtl_stvHysEngBrkReq>"
  BS_Result/7 -> ToWs_Result_Bus_Sig7/1  "<CrCtl_trqLead>"
  BS_Result/8 -> ToWs_Result_Bus_Sig8/1  "<CrCtl_trqLimAct>"
  BS_Result/9 -> ToWs_Result_Bus_Sig9/1  "<CrCtl_trqMin>"
  BS_Result/10 -> ToWs_Result_Bus_Sig10/1  "<CrCtl_trqReq>"
  BS_Result/11 -> ToWs_Result_Bus_Sig11/1  "<CrCtl_trqReqOld>"
  BS_Result/12 -> ToWs_Result_Bus_Sig12/1  "<CrCtl_vMax>"
  specifyOutputs/1(result) -> result/1

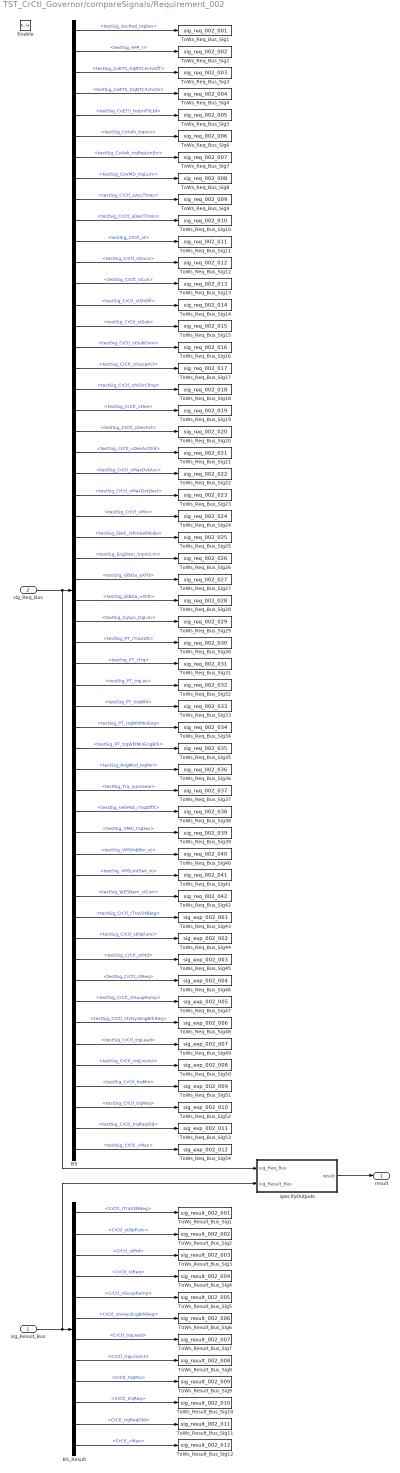
== system TST_CrCtl_Governor/compareSignals/Requirement_002 ==
  sig_Result_Bus : Inport
  sig_Req_Bus : Inport  Port=2
  Enable : EnablePort
  BS : BusSelector  OutputSignals=testSig_AccPed_trqDes,testSig_APP_r,testSig_CoETS_trqNTCActvOff,testSig_CoETS_trqNTCActvOn,testSig_CoETS_trqUnFltLtd,testSig_CoVeh_trqAcs,testSig_CoVeh_trqPrpLimErr,testSig_CoVMD_trqLLim,testSig_CrCtl_aAccThres,testSig_CrCtl_aDeclThres,testSig_CrCtl_st,testSig_CrCtl_stGvnr,testSig_CrCtl_stLck,testSig_CrCtl_stShOff,testSig_CrCtl_stSub,testSig_CrCtl_stSubGvnr,testSig_CrCtl_stSuspAct,testSig_CrCtl_stVDirChng,testSig_CrCtl_vDes,testSig_CrCtl_vDesAct,testSig_CrCtl_vDesActOld,testSig_CrCtl_vMaxDvtAcc,testSig_CrCtl_vMaxDvtDecl,testSig_CrCtl_vMin,testSig_EBrk_stPreSelMode,testSig_EngDem_trqInrLim,testSig_GlbDa_aXFlt,testSig_GlbDa_vXFlt,testSig_InjSys_trqLim,testSig_PT_rTraV2N,testSig_PT_rTrq,testSig_PT_trqLos,testSig_PT_trqWhl,testSig_PT_trqWhlMinEng,testSig_PT_trqWhlMinEngBrk,testSig_RngMod_trqMin,testSig_Tra_numGear,testSig_VehMot_rTrqDfftl,testSig_VMD_trqDes,testSig_VMSAdjBtn_st,testSig_VMSLmtSwt_st,testSig_WESDem_stCurr,testSig_CrCtl_rTraV2NBeg,testSig_CrCtl_stOpFunc,testSig_CrCtl_stPtd,testSig_CrCtl_stReq,testSig_CrCtl_stSuspRamp,testSig_CrCtl_stvHysEngBrkReq,testSig_CrCtl_trqLead,testSig_CrCtl_trqLimAct,testSig_CrCtl_trqMin,testSig_CrCtl_trqReq,testSig_CrCtl_trqReqOld,testSig_CrCtl_vMax
  BS_Result : BusSelector  OutputSignals=CrCtl_rTraV2NBeg,CrCtl_stOpFunc,CrCtl_stPtd,CrCtl_stReq,CrCtl_stSuspRamp,CrCtl_stvHysEngBrkReq,CrCtl_trqLead,CrCtl_trqLimAct,CrCtl_trqMin,CrCtl_trqReq,CrCtl_trqReqOld,CrCtl_vMax
  ToWs_Req_Bus_Sig1 : ToWorkspace  VariableName=sig_req_002_001  SaveFormat=Structure With Time
  ToWs_Req_Bus_Sig10 : ToWorkspace  VariableName=sig_req_002_010  SaveFormat=Structure With Time
  ToWs_Req_Bus_Sig11 : ToWorkspace  VariableName=sig_req_002_011  SaveFormat=Structure With Time
  ToWs_Req_Bus_Sig12 : ToWorkspace  VariableName=sig_req_002_012  SaveFormat=Structure With Time
  ToWs_Req_Bus_Sig13 : ToWorkspace  VariableName=sig_req_002_013  SaveFormat=Structure With Time
  ToWs_Req_Bus_Sig14 : ToWorkspace  VariableName=sig_req_002_014  SaveFormat=Structure With Time
  ToWs_Req_Bus_Sig15 : ToWorkspace  VariableName=sig_req_002_015  SaveFormat=Structure With Time
  ToWs_Req_Bus_Sig16 : ToWorkspace  VariableName=sig_req_002_016  SaveFormat=Structure With Time
  ToWs_Req_Bus_Sig17 : ToWorkspace  VariableName=sig_req_002_017  SaveFormat=Structure With Time
  ToWs_Req_Bus_Sig18 : ToWorkspace  VariableName=sig_req_002_018  SaveFormat=Structure With Time
  ToWs_Req_Bus_Sig19 : ToWorkspace  VariableName=sig_req_002_019  SaveFormat=Structure With Time
  ToWs_Req_Bus_Sig2 : ToWorkspace  VariableName=sig_req_002_002  SaveFormat=Structure With Time
  ToWs_Req_Bus_Sig20 : ToWorkspace  VariableName=sig_req_002_020  SaveFormat=Structure With Time
  ToWs_Req_Bus_Sig21 : ToWorkspace  VariableName=sig_req_002_021  SaveFormat=Structure With Time
  ToWs_Req_Bus_Sig22 : ToWorkspace  VariableName=sig_req_002_022  SaveFormat=Structure With Time
  ToWs_Req_Bus_Sig23 : ToWorkspace  VariableName=sig_req_002_023  SaveFormat=Structure With Time
  ToWs_Req_Bus_Sig24 : ToWorkspace  VariableName=sig_req_002_024  SaveFormat=Structure With Time
  ToWs_Req_Bus_Sig25 : ToWorkspace  VariableName=sig_req_002_025  SaveFormat=Structure With Time
  ToWs_Req_Bus_Sig26 : ToWorkspace  VariableName=sig_req_002_026  SaveFormat=Structure With Time
  ToWs_Req_Bus_Sig27 : ToWorkspace  VariableName=sig_req_002_027  SaveFormat=Structure With Time
  ToWs_Req_Bus_Sig28 : ToWorkspace  VariableName=sig_req_002_028  SaveFormat=Structure With Time
  ToWs_Req_Bus_Sig29 : ToWorkspace  VariableName=sig_req_002_029  SaveFormat=Structure With Time
  ToWs_Req_Bus_Sig3 : ToWorkspace  VariableName=sig_req_002_003  SaveFormat=Structure With Time
  ToWs_Req_Bus_Sig30 : ToWorkspace  VariableName=sig_req_002_030  SaveFormat=Structure With Time
  ToWs_Req_Bus_Sig31 : ToWorkspace  VariableName=sig_req_002_031  SaveFormat=Structure With Time
  ToWs_Req_Bus_Sig32 : ToWorkspace  VariableName=sig_req_002_032  SaveFormat=Structure With Time
  ToWs_Req_Bus_Sig33 : ToWorkspace  VariableName=sig_req_002_033  SaveFormat=Structure With Time
  ToWs_Req_Bus_Sig34 : ToWorkspace  VariableName=sig_req_002_034  SaveFormat=Structure With Time
  ToWs_Req_Bus_Sig35 : ToWorkspace  VariableName=sig_req_002_035  SaveFormat=Structure With Time
  ToWs_Req_Bus_Sig36 : ToWorkspace  VariableName=sig_req_002_036  SaveFormat=Structure With Time
  ToWs_Req_Bus_Sig37 : ToWorkspace  VariableName=sig_req_002_037  SaveFormat=Structure With Time
  ToWs_Req_Bus_Sig38 : ToWorkspace  VariableName=sig_req_002_038  SaveFormat=Structure With Time
  ToWs_Req_Bus_Sig39 : ToWorkspace  VariableName=sig_req_002_039  SaveFormat=Structure With Time
  ToWs_Req_Bus_Sig4 : ToWorkspace  VariableName=sig_req_002_004  SaveFormat=Structure With Time
  ToWs_Req_Bus_Sig40 : ToWorkspace  VariableName=sig_req_002_040  SaveFormat=Structure With Time
  ToWs_Req_Bus_Sig41 : ToWorkspace  VariableName=sig_req_002_041  SaveFormat=Structure With Time
  ToWs_Req_Bus_Sig42 : ToWorkspace  VariableName=sig_req_002_042  SaveFormat=Structure With Time
  ToWs_Req_Bus_Sig43 : ToWorkspace  VariableName=sig_exp_002_001  SaveFormat=Structure With Time
  ToWs_Req_Bus_Sig44 : ToWorkspace  VariableName=sig_exp_002_002  SaveFormat=Structure With Time
  ToWs_Req_Bus_Sig45 : ToWorkspace  VariableName=sig_exp_002_003  SaveFormat=Structure With Time
  ToWs_Req_Bus_Sig46 : ToWorkspace  VariableName=sig_exp_002_004  SaveFormat=Structure With Time
  ToWs_Req_Bus_Sig47 : ToWorkspace  VariableName=sig_exp_002_005  SaveFormat=Structure With Time
  ToWs_Req_Bus_Sig48 : ToWorkspace  VariableName=sig_exp_002_006  SaveFormat=Structure With Time
  ToWs_Req_Bus_Sig49 : ToWorkspace  VariableName=sig_exp_002_007  SaveFormat=Structure With Time
  ToWs_Req_Bus_Sig5 : ToWorkspace  VariableName=sig_req_002_005  SaveFormat=Structure With Time
  ToWs_Req_Bus_Sig50 : ToWorkspace  VariableName=sig_exp_002_008  SaveFormat=Structure With Time
  ToWs_Req_Bus_Sig51 : ToWorkspace  VariableName=sig_exp_002_009  SaveFormat=Structure With Time
  ToWs_Req_Bus_Sig52 : ToWorkspace  VariableName=sig_exp_002_010  SaveFormat=Structure With Time
  ToWs_Req_Bus_Sig53 : ToWorkspace  VariableName=sig_exp_002_011  SaveFormat=Structure With Time
  ToWs_Req_Bus_Sig54 : ToWorkspace  VariableName=sig_exp_002_012  SaveFormat=Structure With Time
  ToWs_Req_Bus_Sig6 : ToWorkspace  VariableName=sig_req_002_006  SaveFormat=Structure With Time
  ToWs_Req_Bus_Sig7 : ToWorkspace  VariableName=sig_req_002_007  SaveFormat=Structure With Time
  ToWs_Req_Bus_Sig8 : ToWorkspace  VariableName=sig_req_002_008  SaveFormat=Structure With Time
  ToWs_Req_Bus_Sig9 : ToWorkspace  VariableName=sig_req_002_009  SaveFormat=Structure With Time
  ToWs_Result_Bus_Sig1 : ToWorkspace  VariableName=sig_result_002_001  SaveFormat=Structure With Time
  ToWs_Result_Bus_Sig10 : ToWorkspace  VariableName=sig_result_002_010  SaveFormat=Structure With Time
  ToWs_Result_Bus_Sig11 : ToWorkspace  VariableName=sig_result_002_011  SaveFormat=Structure With Time
  ToWs_Result_Bus_Sig12 : ToWorkspace  VariableName=sig_result_002_012  SaveFormat=Structure With Time
  ToWs_Result_Bus_Sig2 : ToWorkspace  VariableName=sig_result_002_002  SaveFormat=Structure With Time
  ToWs_Result_Bus_Sig3 : ToWorkspace  VariableName=sig_result_002_003  SaveFormat=Structure With Time
  ToWs_Result_Bus_Sig4 : ToWorkspace  VariableName=sig_result_002_004  SaveFormat=Structure With Time
  ToWs_Result_Bus_Sig5 : ToWorkspace  VariableName=sig_result_002_005  SaveFormat=Structure With Time
  ToWs_Result_Bus_Sig6 : ToWorkspace  VariableName=sig_result_002_006  SaveFormat=Structure With Time
  ToWs_Result_Bus_Sig7 : ToWorkspace  VariableName=sig_result_002_007  SaveFormat=Structure With Time
  ToWs_Result_Bus_Sig8 : ToWorkspace  VariableName=sig_result_002_008  SaveFormat=Structure With Time
  ToWs_Result_Bus_Sig9 : ToWorkspace  VariableName=sig_result_002_009  SaveFormat=Structure With Time
  specifyOutputs : Subsystem
  result : Outport
  wires:
  sig_Req_Bus/1 -> BS/1, specifyOutputs/1(sig_Req_Bus)
  BS/1 -> ToWs_Req_Bus_Sig1/1  "<testSig_AccPed_trqDes>"
  BS/2 -> ToWs_Req_Bus_Sig2/1  "<testSig_APP_r>"
  BS/3 -> ToWs_Req_Bus_Sig3/1  "<testSig_CoETS_trqNTCActvOff>"
  BS/4 -> ToWs_Req_Bus_Sig4/1  "<testSig_CoETS_trqNTCActvOn>"
  BS/5 -> ToWs_Req_Bus_Sig5/1  "<testSig_CoETS_trqUnFltLtd>"
  BS/6 -> ToWs_Req_Bus_Sig6/1  "<testSig_CoVeh_trqAcs>"
  BS/7 -> ToWs_Req_Bus_Sig7/1  "<testSig_CoVeh_trqPrpLimErr>"
  BS/8 -> ToWs_Req_Bus_Sig8/1  "<testSig_CoVMD_trqLLim>"
  BS/9 -> ToWs_Req_Bus_Sig9/1  "<testSig_CrCtl_aAccThres>"
  BS/10 -> ToWs_Req_Bus_Sig10/1  "<testSig_CrCtl_aDeclThres>"
  BS/11 -> ToWs_Req_Bus_Sig11/1  "<testSig_CrCtl_st>"
  BS/12 -> ToWs_Req_Bus_Sig12/1  "<testSig_CrCtl_stGvnr>"
  BS/13 -> ToWs_Req_Bus_Sig13/1  "<testSig_CrCtl_stLck>"
  BS/14 -> ToWs_Req_Bus_Sig14/1  "<testSig_CrCtl_stShOff>"
  BS/15 -> ToWs_Req_Bus_Sig15/1  "<testSig_CrCtl_stSub>"
  BS/16 -> ToWs_Req_Bus_Sig16/1  "<testSig_CrCtl_stSubGvnr>"
  BS/17 -> ToWs_Req_Bus_Sig17/1  "<testSig_CrCtl_stSuspAct>"
  BS/18 -> ToWs_Req_Bus_Sig18/1  "<testSig_CrCtl_stVDirChng>"
  BS/19 -> ToWs_Req_Bus_Sig19/1  "<testSig_CrCtl_vDes>"
  BS/20 -> ToWs_Req_Bus_Sig20/1  "<testSig_CrCtl_vDesAct>"
  BS/21 -> ToWs_Req_Bus_Sig21/1  "<testSig_CrCtl_vDesActOld>"
  BS/22 -> ToWs_Req_Bus_Sig22/1  "<testSig_CrCtl_vMaxDvtAcc>"
  BS/23 -> ToWs_Req_Bus_Sig23/1  "<testSig_CrCtl_vMaxDvtDecl>"
  BS/24 -> ToWs_Req_Bus_Sig24/1  "<testSig_CrCtl_vMin>"
  BS/25 -> ToWs_Req_Bus_Sig25/1  "<testSig_EBrk_stPreSelMode>"
  BS/26 -> ToWs_Req_Bus_Sig26/1  "<testSig_EngDem_trqInrLim>"
  BS/27 -> ToWs_Req_Bus_Sig27/1  "<testSig_GlbDa_aXFlt>"
  BS/28 -> ToWs_Req_Bus_Sig28/1  "<testSig_GlbDa_vXFlt>"
  BS/29 -> ToWs_Req_Bus_Sig29/1  "<testSig_InjSys_trqLim>"
  BS/30 -> ToWs_Req_Bus_Sig30/1  "<testSig_PT_rTraV2N>"
  BS/31 -> ToWs_Req_Bus_Sig31/1  "<testSig_PT_rTrq>"
  BS/32 -> ToWs_Req_Bus_Sig32/1  "<testSig_PT_trqLos>"
  BS/33 -> ToWs_Req_Bus_Sig33/1  "<testSig_PT_trqWhl>"
  BS/34 -> ToWs_Req_Bus_Sig34/1  "<testSig_PT_trqWhlMinEng>"
  BS/35 -> ToWs_Req_Bus_Sig35/1  "<testSig_PT_trqWhlMinEngBrk>"
  BS/36 -> ToWs_Req_Bus_Sig36/1  "<testSig_RngMod_trqMin>"
  BS/37 -> ToWs_Req_Bus_Sig37/1  "<testSig_Tra_numGear>"
  BS/38 -> ToWs_Req_Bus_Sig38/1  "<testSig_VehMot_rTrqDfftl>"
  BS/39 -> ToWs_Req_Bus_Sig39/1  "<testSig_VMD_trqDes>"
  BS/40 -> ToWs_Req_Bus_Sig40/1  "<testSig_VMSAdjBtn_st>"
  BS/41 -> ToWs_Req_Bus_Sig41/1  "<testSig_VMSLmtSwt_st>"
  BS/42 -> ToWs_Req_Bus_Sig42/1  "<testSig_WESDem_stCurr>"
  BS/43 -> ToWs_Req_Bus_Sig43/1  "<testSig_CrCtl_rTraV2NBeg>"
  BS/44 -> ToWs_Req_Bus_Sig44/1  "<testSig_CrCtl_stOpFunc>"
  BS/45 -> ToWs_Req_Bus_Sig45/1  "<testSig_CrCtl_stPtd>"
  BS/46 -> ToWs_Req_Bus_Sig46/1  "<testSig_CrCtl_stReq>"
  BS/47 -> ToWs_Req_Bus_Sig47/1  "<testSig_CrCtl_stSuspRamp>"
  BS/48 -> ToWs_Req_Bus_Sig48/1  "<testSig_CrCtl_stvHysEngBrkReq>"
  BS/49 -> ToWs_Req_Bus_Sig49/1  "<testSig_CrCtl_trqLead>"
  BS/50 -> ToWs_Req_Bus_Sig50/1  "<testSig_CrCtl_trqLimAct>"
  BS/51 -> ToWs_Req_Bus_Sig51/1  "<testSig_CrCtl_trqMin>"
  BS/52 -> ToWs_Req_Bus_Sig52/1  "<testSig_CrCtl_trqReq>"
  BS/53 -> ToWs_Req_Bus_Sig53/1  "<testSig_CrCtl_trqReqOld>"
  BS/54 -> ToWs_Req_Bus_Sig54/1  "<testSig_CrCtl_vMax>"
  sig_Result_Bus/1 -> BS_Result/1, specifyOutputs/2(sig_Result_Bus)
  BS_Result/1 -> ToWs_Result_Bus_Sig1/1  "<CrCtl_rTraV2NBeg>"
  BS_Result/2 -> ToWs_Result_Bus_Sig2/1  "<CrCtl_stOpFunc>"
  BS_Result/3 -> ToWs_Result_Bus_Sig3/1  "<CrCtl_stPtd>"
  BS_Result/4 -> ToWs_Result_Bus_Sig4/1  "<CrCtl_stReq>"
  BS_Result/5 -> ToWs_Result_Bus_Sig5/1  "<CrCtl_stSuspRamp>"
  BS_Result/6 -> ToWs_Result_Bus_Sig6/1  "<CrCtl_stvHysEngBrkReq>"
  BS_Result/7 -> ToWs_Result_Bus_Sig7/1  "<CrCtl_trqLead>"
  BS_Result/8 -> ToWs_Result_Bus_Sig8/1  "<CrCtl_trqLimAct>"
  BS_Result/9 -> ToWs_Result_Bus_Sig9/1  "<CrCtl_trqMin>"
  BS_Result/10 -> ToWs_Result_Bus_Sig10/1  "<CrCtl_trqReq>"
  BS_Result/11 -> ToWs_Result_Bus_Sig11/1  "<CrCtl_trqReqOld>"
  BS_Result/12 -> ToWs_Result_Bus_Sig12/1  "<CrCtl_vMax>"
  specifyOutputs/1(result) -> result/1
